simulink model "MultiAgentMaths"  (R2017a)
settings: Solver=ode23t  StartTime=0.0  StopTime=5  FixedStep=tstep  MaxStep=tstep  RelTol=1e-3
InitFcn:
  | initSim;
StopFcn:
  | plotSimSolution;
values from neighbouring files (symbols this model uses):
  tstep = 0.01    [initSim.m]
undefined symbols (not defined in the file or in its folder): m
settings Model: Creator=yn15  LastModifiedBy=daw15
settings OptimizationCC: LifeSpan=inf
settings DebuggingCC: SFUnexpectedBacktrackingDiag=warning  SFNoUnconditionalDefaultTransitionDiag=warning  SFExecutionAtInitializationDiag=none
settings GRTTargetCC: TargetLangStandard=C89/C90 (ANSI)
settings ConfigComp: CovMetricSettings=dw  CovHtmlReporting=on  CovSaveCumulativeToWorkspaceVar=on  CovSaveSingleToWorkspaceVar=on  CovExternalEMLEnable=off

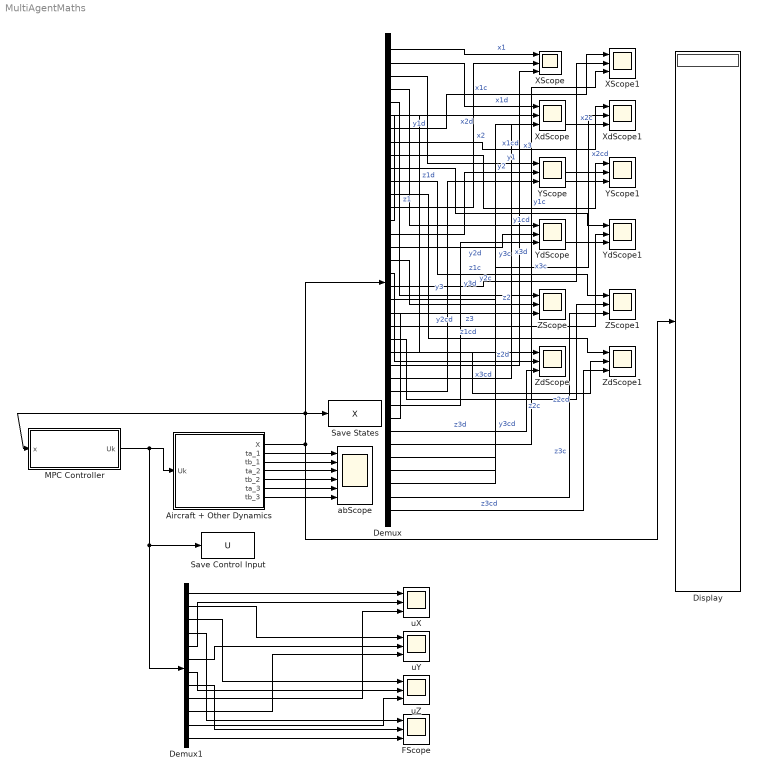
== system MultiAgentMaths ==
  Aircraft + Other Dynamics : Subsystem
  Demux : Demux  Outputs=36
  Demux1 : Demux  Outputs=12
  Display : Display
  FScope : Scope  NumInputPorts=3
  "MPC Controller " : Subsystem
  Save Control Input : ToWorkspace  VariableName=U  SampleTime=-1
      settings: Save2DSignal=2-D array (concatenate along first dimension)
  Save States : ToWorkspace  VariableName=X  SaveFormat=Timeseries  SampleTime=-1
  XScope : Scope  NumInputPorts=3
  XScope1 : Scope  NumInputPorts=3
  XdScope : Scope  NumInputPorts=3
  XdScope1 : Scope  NumInputPorts=3
  YScope : Scope  NumInputPorts=3
  YScope1 : Scope  NumInputPorts=3
  YdScope : Scope  NumInputPorts=3
  YdScope1 : Scope  NumInputPorts=3
  ZScope : Scope  NumInputPorts=3
  ZScope1 : Scope  NumInputPorts=3
  ZdScope : Scope  NumInputPorts=3
  ZdScope1 : Scope  NumInputPorts=3
  abScope : Scope  NumInputPorts=6
  uX : Scope  NumInputPorts=3
  uY : Scope  NumInputPorts=3
  uZ : Scope  NumInputPorts=3
  wires:
  Aircraft + Other Dynamics/1(X) -> Save States/1, "MPC Controller "/1(x), Demux/1, Display/1
  "MPC Controller "/1(Uk) -> Demux1/1, Save Control Input/1, Aircraft + Other Dynamics/1(Uk)
  Aircraft + Other Dynamics/2(ta_1) -> abScope/1
  Aircraft + Other Dynamics/3(tb_1) -> abScope/2
  Aircraft + Other Dynamics/4(ta_2) -> abScope/3
  Aircraft + Other Dynamics/5(tb_2) -> abScope/4
  Aircraft + Other Dynamics/6(ta_3) -> abScope/5
  Aircraft + Other Dynamics/7(tb_3) -> abScope/6
  Demux1/1 -> uX/1
  Demux1/2 -> uY/1
  Demux1/3 -> uZ/1
  Demux1/4 -> FScope/1
  Demux1/5 -> uX/2
  Demux1/6 -> uY/2
  Demux1/7 -> uZ/2
  Demux1/8 -> FScope/2
  Demux1/9 -> uX/3
  Demux1/10 -> uY/3
  Demux1/11 -> uZ/3
  Demux1/12 -> FScope/3
  Demux/1 -> XScope/1  "x1"
  Demux/2 -> XdScope/1  "x1d"
  Demux/3 -> YScope/1  "y1"
  Demux/4 -> YdScope/1  "y1d"
  Demux/5 -> ZScope/1  "z1"
  Demux/6 -> ZdScope/1  "z1d"
  Demux/7 -> XScope1/1  "x1c"
  Demux/8 -> XdScope1/1  "x1cd"
  Demux/9 -> YScope1/1  "y1c"
  Demux/10 -> YdScope1/1  "y1cd"
  Demux/11 -> ZScope1/1  "z1c"
  Demux/12 -> ZdScope1/1  "z1cd"
  Demux/13 -> XScope/2  "x2"
  Demux/14 -> XdScope/2  "x2d"
  Demux/15 -> YScope/2  "y2"
  Demux/16 -> YdScope/2  "y2d"
  Demux/17 -> ZScope/2  "z2"
  Demux/18 -> ZdScope/2  "z2d"
  Demux/19 -> XScope1/2  "x2c"
  Demux/20 -> XdScope1/2  "x2cd"
  Demux/21 -> YScope1/2  "y2c"
  Demux/22 -> YdScope1/2  "y2cd"
  Demux/23 -> ZScope1/2  "z2c"
  Demux/24 -> ZdScope1/2  "z2cd"
  Demux/25 -> XScope/3  "x3"
  Demux/26 -> XdScope/3  "x3d"
  Demux/27 -> YScope/3  "y3"
  Demux/28 -> YdScope/3  "y3d"
  Demux/29 -> ZScope/3  "z3"
  Demux/30 -> ZdScope/3  "z3d"
  Demux/31 -> XScope1/3  "x3c"
  Demux/32 -> XdScope1/3  "x3cd"
  Demux/33 -> YScope1/3  "y3c"
  Demux/34 -> YdScope1/3  "y3cd"
  Demux/35 -> ZScope1/3  "z3c"
  Demux/36 -> ZdScope1/3  "z3cd"

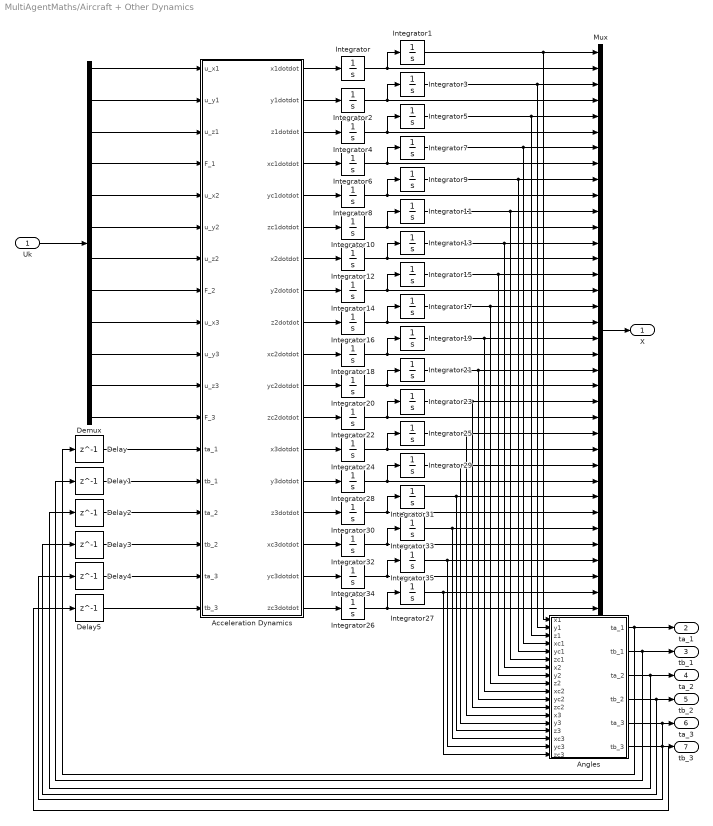
== system MultiAgentMaths/Aircraft + Other Dynamics ==
  Uk : Inport
  Acceleration Dynamics : MATLAB Function  TreatAsAtomicUnit=on
  Angles : MATLAB Function  TreatAsAtomicUnit=on
  Delay{,1..5} (6 alike) : Delay  DelayLength=1  SampleTime=tstep
  Demux : Demux  Outputs=12
  Integrator{,2..4,6,8..10,12,14..16,18,20..22,24,26,28..30,32,34..35} (24 alike) : Integrator
  Integrator1 : Integrator  InitialCondition=2.1
  Integrator11 : Integrator  InitialCondition=1
  Integrator13 : Integrator  InitialCondition=3
  Integrator17 : Integrator  InitialCondition=2.2
  Integrator19 : Integrator  InitialCondition=3
  Integrator23 : Integrator  InitialCondition=1
  Integrator25 : Integrator  InitialCondition=3.9
  Integrator27 : Integrator  InitialCondition=1
  Integrator31 : Integrator  InitialCondition=2.2
  Integrator33 : Integrator  InitialCondition=3.9
  Integrator5 : Integrator  InitialCondition=2.2
  Integrator7 : Integrator  InitialCondition=2.1
  Mux : Mux  Inputs=36
  X : Outport
  ta_1 : Outport  Port=2
  tb_1 : Outport  Port=3
  ta_2 : Outport  Port=4
  tb_2 : Outport  Port=5
  ta_3 : Outport  Port=6
  tb_3 : Outport  Port=7
  wires:
  Integrator/1 -> Mux/2, Integrator1/1
  Integrator2/1 -> Mux/4, Integrator3/1
  Integrator4/1 -> Mux/6, Integrator5/1
  Integrator6/1 -> Mux/8, Integrator7/1
  Integrator8/1 -> Mux/10, Integrator9/1
  Integrator10/1 -> Mux/12, Integrator11/1
  Integrator12/1 -> Mux/14, Integrator13/1
  Integrator14/1 -> Mux/16, Integrator15/1
  Integrator16/1 -> Mux/18, Integrator17/1
  Integrator18/1 -> Mux/20, Integrator19/1
  Integrator20/1 -> Mux/22, Integrator21/1
  Integrator22/1 -> Mux/24, Integrator23/1
  Integrator1/1 -> Mux/1, Angles/1(x1)
  Integrator3/1 -> Mux/3, Angles/2(y1)
  Integrator5/1 -> Mux/5, Angles/3(z1)
  Integrator7/1 -> Angles/4(xc1), Mux/7
  Integrator9/1 -> Mux/9, Angles/5(yc1)
  Integrator11/1 -> Mux/11, Angles/6(zc1)
  Integrator13/1 -> Mux/13, Angles/7(x2)
  Integrator15/1 -> Mux/15, Angles/8(y2)
  Integrator17/1 -> Mux/17, Angles/9(z2)
  Integrator19/1 -> Angles/10(xc2), Mux/19
  Integrator21/1 -> Mux/21, Angles/11(yc2)
  Integrator23/1 -> Mux/23, Angles/12(zc2)
  Mux/1 -> X/1
  Uk/1 -> Demux/1
  Demux/12 -> Acceleration Dynamics/12(F_3)
  Angles/1(ta_1) -> ta_1/1, Delay/1
  Angles/2(tb_1) -> Delay1/1, tb_1/1
  Delay/1 -> Acceleration Dynamics/13(ta_1)
  Delay1/1 -> Acceleration Dynamics/14(tb_1)
  Delay2/1 -> Acceleration Dynamics/15(ta_2)
  Delay3/1 -> Acceleration Dynamics/16(tb_2)
  Delay4/1 -> Acceleration Dynamics/17(ta_3)
  Delay5/1 -> Acceleration Dynamics/18(tb_3)
  Angles/3(ta_2) -> Delay2/1, ta_2/1
  Angles/4(tb_2) -> Delay3/1, tb_2/1
  Angles/5(ta_3) -> ta_3/1, Delay4/1
  Angles/6(tb_3) -> Delay5/1, tb_3/1
  Demux/1 -> Acceleration Dynamics/1(u_x1)
  Demux/2 -> Acceleration Dynamics/2(u_y1)
  Demux/3 -> Acceleration Dynamics/3(u_z1)
  Demux/4 -> Acceleration Dynamics/4(F_1)
  Demux/5 -> Acceleration Dynamics/5(u_x2)
  Demux/6 -> Acceleration Dynamics/6(u_y2)
  Demux/7 -> Acceleration Dynamics/7(u_z2)
  Demux/8 -> Acceleration Dynamics/8(F_2)
  Demux/9 -> Acceleration Dynamics/9(u_x3)
  Demux/10 -> Acceleration Dynamics/10(u_y3)
  Demux/11 -> Acceleration Dynamics/11(u_z3)
  Integrator29/1 -> Angles/14(y3), Mux/27
  Integrator30/1 -> Mux/30, Integrator31/1
  Integrator24/1 -> Integrator25/1, Mux/26
  Integrator26/1 -> Integrator27/1, Mux/36
  Integrator31/1 -> Angles/15(z3), Mux/29
  Integrator33/1 -> Angles/16(xc3), Mux/31
  Integrator28/1 -> Mux/28, Integrator29/1
  Integrator25/1 -> Mux/25, Angles/13(x3)
  Integrator32/1 -> Mux/32, Integrator33/1
  Integrator34/1 -> Mux/34, Integrator35/1
  Integrator35/1 -> Angles/17(yc3), Mux/33
  Integrator27/1 -> Angles/18(zc3), Mux/35
  Acceleration Dynamics/1(x1dotdot) -> Integrator/1
  Acceleration Dynamics/2(y1dotdot) -> Integrator2/1
  Acceleration Dynamics/3(z1dotdot) -> Integrator4/1
  Acceleration Dynamics/4(xc1dotdot) -> Integrator6/1
  Acceleration Dynamics/5(yc1dotdot) -> Integrator8/1
  Acceleration Dynamics/6(zc1dotdot) -> Integrator10/1
  Acceleration Dynamics/7(x2dotdot) -> Integrator12/1
  Acceleration Dynamics/8(y2dotdot) -> Integrator14/1
  Acceleration Dynamics/9(z2dotdot) -> Integrator16/1
  Acceleration Dynamics/10(xc2dotdot) -> Integrator18/1
  Acceleration Dynamics/11(yc2dotdot) -> Integrator20/1
  Acceleration Dynamics/12(zc2dotdot) -> Integrator22/1
  Acceleration Dynamics/13(x3dotdot) -> Integrator24/1
  Acceleration Dynamics/14(y3dotdot) -> Integrator28/1
  Acceleration Dynamics/15(z3dotdot) -> Integrator30/1
  Acceleration Dynamics/16(xc3dotdot) -> Integrator32/1
  Acceleration Dynamics/17(yc3dotdot) -> Integrator34/1
  Acceleration Dynamics/18(zc3dotdot) -> Integrator26/1

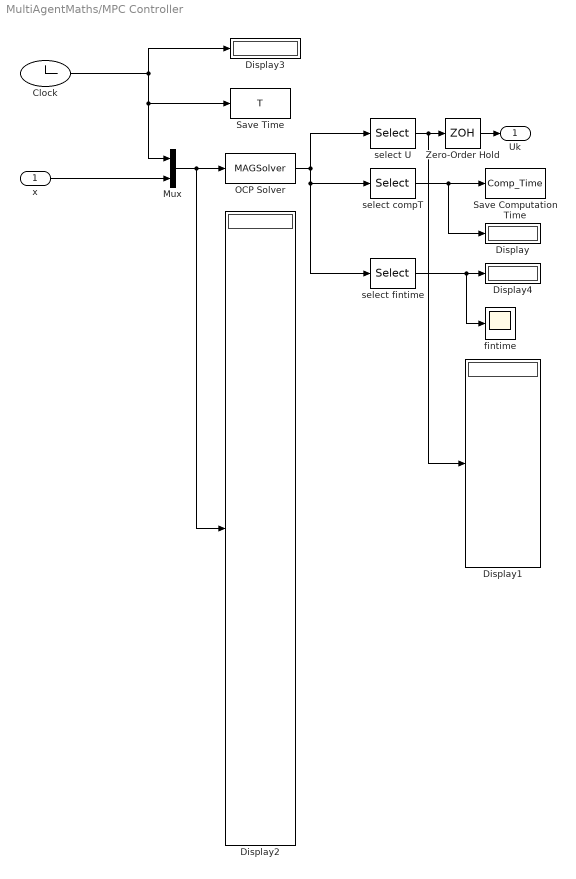
== system MultiAgentMaths/MPC Controller  ==
  x : Inport
  Clock : Clock
  Display{,1..4} (5 alike) : Display
  Mux : Mux  Inputs=2
  OCP Solver : MATLABFcn  MATLABFcn=MAGSolver  OutputDimensions=m+2
  "Save Computation Time " : ToWorkspace  VariableName=Comp_Time  SampleTime=tstep
      settings: Save2DSignal=2-D array (concatenate along first dimension)
  Save Time : ToWorkspace  VariableName=T  SampleTime=-1
      settings: Save2DSignal=2-D array (concatenate along first dimension)
  Zero-Order Hold : ZeroOrderHold  SampleTime=tstep
  fintime : Scope
  select U : Selector  IndexOptions=Index vector (dialog)  Indices=3:m+2  OutputSizes=1
  select compT : Selector  IndexOptions=Index vector (dialog)  Indices=2  OutputSizes=1
  select fintime : Selector  IndexOptions=Index vector (dialog)  Indices=1  OutputSizes=1
  Uk : Outport
  wires:
  select U/1 -> Zero-Order Hold/1, Display1/1
  Clock/1 -> Save Time/1, Mux/1, Display3/1
  select compT/1 -> Display/1, "Save Computation Time "/1
  Mux/1 -> Display2/1, OCP Solver/1
  x/1 -> Mux/2
  select fintime/1 -> fintime/1, Display4/1
  OCP Solver/1 -> select U/1, select fintime/1, select compT/1
  Zero-Order Hold/1 -> Uk/1

== matlab function MultiAgentMaths/Aircraft + Other Dynamics/Angles ==
  data: x1 input; ta_1 output; y1 input; z1 input; xc1 input; yc1 input; zc1 input; tb_1 output; x2 input; y2 input; z2 input; xc2 input; yc2 input; zc2 input; x3 input; y3 input; z3 input; ta_2 output; tb_2 output; ta_3 output; tb_3 output; xc3 input; yc3 input; zc3 input
function [ta_1,tb_1,ta_2,tb_2,ta_3,tb_3] = updateAngles(x1,y1,z1,xc1,yc1,zc1,x2,y2,z2,xc2,yc2,zc2,x3,y3,z3,xc3,yc3,zc3)

ta_1 = (x1-xc1)/(z1-zc1);
tb_1 = (y1-yc1)/(z1-zc1);
ta_2 = (x2-xc2)/(z2-zc2);
tb_2 = (y2-yc2)/(z2-zc2);
ta_3 = (x3-xc3)/(z3-zc3);
tb_3 = (y3-yc3)/(z3-zc3);

== matlab function MultiAgentMaths/Aircraft + Other Dynamics/Acceleration Dynamics ==
  data: x1dotdot output; u_x1 input; u_y1 input; u_z1 input; F_1 input; u_x2 input; u_y2 input; u_z2 input; F_2 input; u_x3 input; u_y3 input; u_z3 input; F_3 input; ta_1 input; tb_1 input; ta_2 input; tb_2 input; ta_3 input; tb_3 input; y1dotdot output; z1dotdot output; xc1dotdot output; yc1dotdot output; zc1dotdot output; x2dotdot output; y2dotdot output; z2dotdot output; xc2dotdot output; yc2dotdot output; zc2dotdot output; x3dotdot output; y3dotdot output; z3dotdot output; xc3dotdot output; yc3dotdot output; zc3dotdot output
function [x1dotdot,y1dotdot,z1dotdot,...
    xc1dotdot,yc1dotdot,zc1dotdot,...
    x2dotdot,y2dotdot,z2dotdot,...
    xc2dotdot,yc2dotdot,zc2dotdot,...
    x3dotdot,y3dotdot,z3dotdot,...
    xc3dotdot,yc3dotdot,zc3dotdot]= fcn(u_x1,u_y1,u_z1,F_1,u_x2,u_y2,u_z2,F_2,u_x3,u_y3,u_z3,F_3,ta_1,tb_1,ta_2,tb_2,ta_3,tb_3)

m_ag = 0.81;
m_pl = 2;
g = 9.81;

x1dotdot = (1/m_ag)*(u_x1 - F_1*(ta_1)); %x1..
y1dotdot = (1/m_ag)*(u_y1 - F_1*(tb_1)); %y1..
z1dotdot = (1/m_ag)*(u_z1 - F_1 - m_ag*g); %z1..
x2dotdot = (1/m_ag)*(u_x2 - F_2*(ta_2)); %x2..
y2dotdot = (1/m_ag)*(u_y2 - F_2*(tb_2)); %y2..
z2dotdot = (1/m_ag)*(u_z2 - F_2 - m_ag*g); %z2..
x3dotdot = (1/m_ag)*(u_x3 - F_3*(ta_3)); %x3..
y3dotdot = (1/m_ag)*(u_y3 - F_3*(tb_3)); %y3..
z3dotdot = (1/m_ag)*(u_z3 - F_3 - m_ag*g); %z3..
xc1dotdot =  (1/m_pl)*(F_1.*ta_1+F_2.*ta_2+F_3.*ta_3);%xcom..
yc1dotdot =  (1/m_pl)*(F_1.*tb_1+F_2.*tb_2+F_3.*tb_3);%ycom..
zc1dotdot =  (1/m_pl)*(F_1+F_2+F_3 - m_pl.*g);%zcom..
xc2dotdot = xc1dotdot;
yc2dotdot = yc1dotdot;
zc2dotdot = zc1dotdot;
xc3dotdot = xc1dotdot;
yc3dotdot = yc1dotdot;
zc3dotdot = zc1dotdot;
